simulink model "TPS_SWC"  (R2023a)
settings: Solver=FixedStepDiscrete  StartTime=0.0  StopTime=10.0  FixedStep=0.1  RelTol=1e-3
settings Model: Creator=eslam  LastModifiedBy=eslam

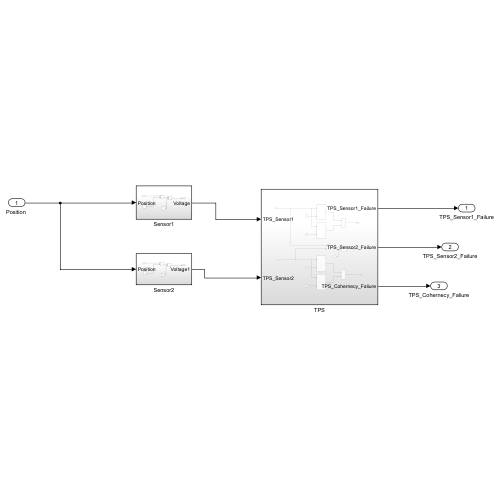
[thumbnail: Simulink's stored preview of the top-level diagram]
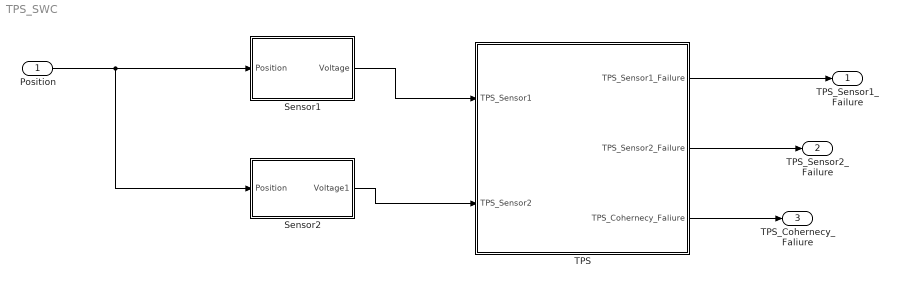
== system TPS_SWC ==
  "Position " : Inport
  Sensor1 : Subsystem
  Sensor2 : Subsystem
  TPS : Subsystem
  TPS_Sensor1_Failure : Outport
  TPS_Sensor2_Failure : Outport  Port=2
  TPS_Cohernecy_Faliure : Outport  Port=3
  wires:
  Sensor1/1(Voltage) -> TPS/1(TPS_Sensor1)
  "Position "/1 -> Sensor1/1(Position), Sensor2/1(Position)
  Sensor2/1(Voltage1) -> TPS/2(TPS_Sensor2)
  TPS/1(TPS_Sensor1_Failure) -> TPS_Sensor1_Failure/1
  TPS/2(TPS_Sensor2_Failure) -> TPS_Sensor2_Failure/1
  TPS/3(TPS_Cohernecy_Faliure) -> TPS_Cohernecy_Faliure/1

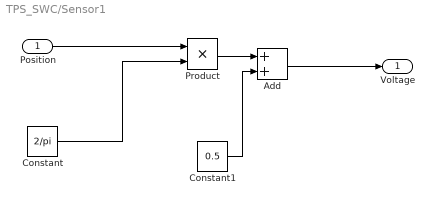
== system TPS_SWC/Sensor1 ==
  Position : Inport
  Add : Sum  AccumDataTypeStr=single
  Constant : Constant  Value=2/pi
  Constant1 : Constant  Value=0.5  OutDataTypeStr=single
  Product : Product  OutDataTypeStr=single
  Voltage : Outport
  wires:
  Position/1 -> Product/1
  Add/1 -> Voltage/1
  Constant1/1 -> Add/2
  Constant/1 -> Product/2
  Product/1 -> Add/1

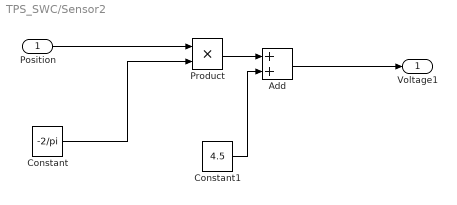
== system TPS_SWC/Sensor2 ==
  Position : Inport
  Add : Sum
  Constant : Constant  Value=-2/pi  OutDataTypeStr=single
  Constant1 : Constant  Value=4.5  OutDataTypeStr=single
  Product : Product
  Voltage1 : Outport
  wires:
  Constant/1 -> Product/2
  Add/1 -> Voltage1/1
  Product/1 -> Add/1
  Position/1 -> Product/1
  Constant1/1 -> Add/2

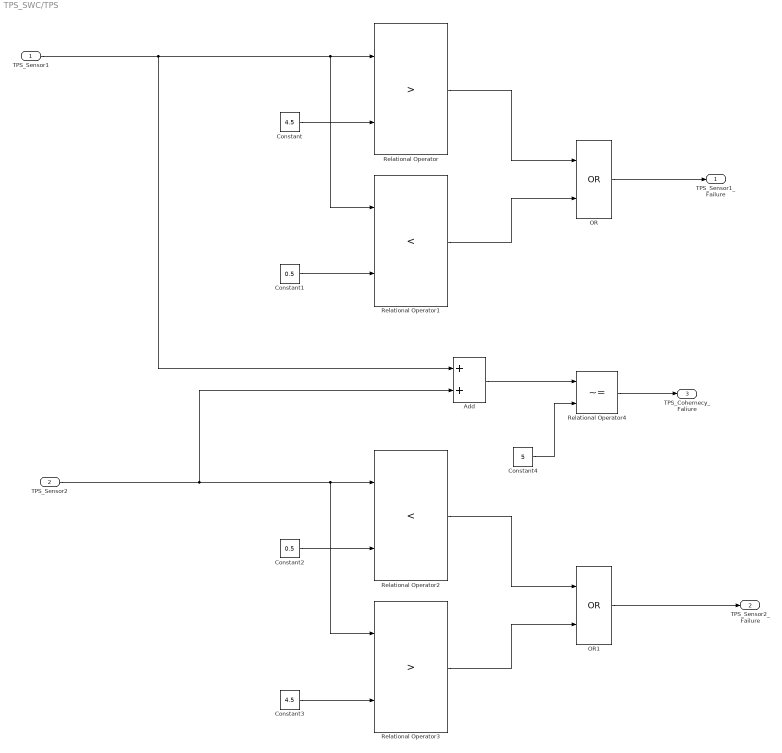
== system TPS_SWC/TPS ==
  TPS_Sensor1 : Inport  OutDataTypeStr=single
  TPS_Sensor2 : Inport  Port=2  OutDataTypeStr=single
  Add : Sum
  Constant : Constant  Value=4.5
  Constant1 : Constant  Value=0.5
  Constant2 : Constant  Value=0.5
  Constant3 : Constant  Value=4.5
  Constant4 : Constant  Value=5
  OR : Logic  Operator=OR  AllPortsSameDT=off  OutDataTypeStr=boolean
  OR1 : Logic  Operator=OR  AllPortsSameDT=off  OutDataTypeStr=boolean
  Relational Operator : RelationalOperator  Operator=>  OutDataTypeStr=boolean  RndMeth=Simplest  InputSameDT=off
  Relational Operator1 : RelationalOperator  Operator=<  OutDataTypeStr=boolean  RndMeth=Simplest  InputSameDT=off
  Relational Operator2 : RelationalOperator  Operator=<  OutDataTypeStr=boolean  RndMeth=Simplest  InputSameDT=off
  Relational Operator3 : RelationalOperator  Operator=>  OutDataTypeStr=boolean  RndMeth=Simplest  InputSameDT=off
  Relational Operator4 : RelationalOperator  Operator=~=  OutDataTypeStr=boolean  RndMeth=Simplest  InputSameDT=off
  TPS_Sensor1_Failure : Outport  OutDataTypeStr=boolean
  TPS_Sensor2_Failure : Outport  Port=2  OutDataTypeStr=boolean
  TPS_Cohernecy_Faliure : Outport  Port=3  OutDataTypeStr=boolean
  wires:
  Constant/1 -> Relational Operator/2
  OR/1 -> TPS_Sensor1_Failure/1
  Relational Operator/1 -> OR/1
  Constant1/1 -> Relational Operator1/2
  Relational Operator1/1 -> OR/2
  TPS_Sensor1/1 -> Add/1, Relational Operator1/1, Relational Operator/1
  Constant3/1 -> Relational Operator3/2
  Constant2/1 -> Relational Operator2/2
  Relational Operator2/1 -> OR1/1
  TPS_Sensor2/1 -> Add/2, Relational Operator3/1, Relational Operator2/1
  Relational Operator3/1 -> OR1/2
  OR1/1 -> TPS_Sensor2_Failure/1
  Add/1 -> Relational Operator4/1
  Constant4/1 -> Relational Operator4/2
  Relational Operator4/1 -> TPS_Cohernecy_Faliure/1
